simulink library "pump"  (R2018a)
settings: Solver=VariableStepAuto  StartTime=0.0  StopTime=10.0  RelTol=1e-3
libraries: fl_lib x3, nesl_utility x2
settings Model: Creator=ChLan  LastModifiedBy=ChLan

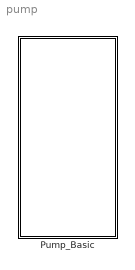
== system pump ==
  Pump_Basic : Subsystem

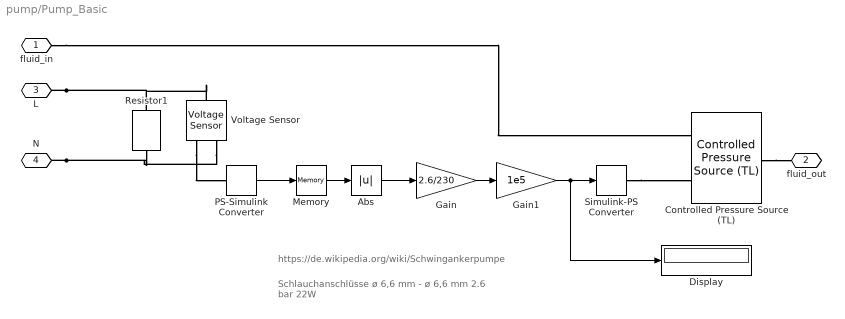
== system pump/Pump_Basic ==
  note: Schlauchanschlüsse ø 6,6 mm - ø 6,6 mm
      | 2.6 bar
      | 22W
  note: https://de.wikipedia.org/wiki/Schwingankerpumpe
  Abs : Abs
  Controlled Pressure Source (TL) : fl_lib/Thermal Liquid/Sources/Controlled Pressure Source (TL)  area=pi*((3.3)^2) mm^2  length=0.02 m  mdot_A_specify=off  mdot_A_priority=None  mdot_A=1 kg/s  mdot_A_nominal_specify=off  mdot_A_nominal_unit=kg/s  mdot_A_nominal_value=1
      settings: SourceProductName=Simscape  SourceProductBaseCode=SS
  Display : Display
  Gain : Gain  Gain=2.6/230
  Gain1 : Gain  Gain=1e5
  Memory : Memory
  PS-Simulink Converter : nesl_utility/PS-Simulink Converter  PhysicalDomain=network_engine_domain  SubClassName=ps_output  LeftPortType=input  RightPortType=output  PseudoPeriodic=off  Frequencies=[]  Unit=1  AffineConversion=off
  Resistor1 : fl_lib/Electrical/Electrical Elements/Resistor  R=2.4 kOhm  i_specify=off  i_priority=None  i=0 A  i_nominal_specify=off  i_nominal_unit=A  i_nominal_value=1  v_specify=off  v_priority=None  v=0 V  v_nominal_specify=off  v_nominal_unit=V  v_nominal_value=1
  Simulink-PS Converter : nesl_utility/Simulink-PS Converter  PhysicalDomain=network_engine_domain  SubClassName=ps_input  LeftPortType=input  RightPortType=output  PseudoPeriodic=off  Frequencies=[]  NoiseDistribution=none  NoiseParameters=[]  Unit=Pa  AffineConversion=off  FilteringAndDerivatives=zero  SimscapeFilterOrder=1  InputFilterTimeConstant=0.001  UdotUserProvided=0
  Voltage Sensor : fl_lib/Electrical/Electrical Sensors/Voltage Sensor
  fluid_in : PMIOPort  Side=Left
  fluid_out : PMIOPort  Port=2  Side=Right
  L : PMIOPort  Port=3  Side=Left
  N : PMIOPort  Port=4  Side=Right
  wires:
  Abs/1 -> Gain/1
  Gain1/1 -> Simulink-PS Converter/1, Display/1
  Gain/1 -> Gain1/1
  Memory/1 -> Abs/1
  PS-Simulink Converter/1 -> Memory/1
  connections:
  Voltage Sensor/RConn1 -- PS-Simulink Converter/LConn1
  L/RConn1 -- Resistor1/LConn1 -- Voltage Sensor/LConn1
  Simulink-PS Converter/RConn1 -- Controlled Pressure Source (TL)/LConn2
  N/RConn1 -- Resistor1/RConn1 -- Voltage Sensor/RConn2
  fluid_in/RConn1 -- Controlled Pressure Source (TL)/LConn1
  Controlled Pressure Source (TL)/RConn1 -- fluid_out/RConn1
